simulink model "untitled1"  (R2019b)
settings: Solver=VariableStepAuto  StartTime=0.0  StopTime=10.0  RelTol=1e-3
libraries: neural x1015
(part 3 of 13)

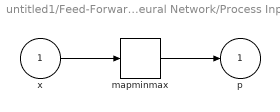
== system untitled1/Feed-Forward Neural Network/Process Input 1 ==
  x : Inport  PortDimensions=1001  SampleTime=0.1
      mask Display: e = 0.06;c1 = [120 230 180]/255;c2 = ([120 230 180]+0)/(256+128);c3 = ([120 230 180]+128)/(256+128);patch([0 1 1 0],[0 0 1 1],c1);patch([0 1 1 1-e 1-e 0+e],[0 0 1 1-e 0+e 0+e],c2);patch([0 0 1 1-e 0+e 0+e],[0 1 1 1-e 1-e 0+e],c3);plot([0 1 1 0 0],[0 0 1 1 0]);
  mapminmax : neural/Processing Functions/mapminmax  xmin=[2.22144146907918305089424393373;1.69636663439423740484812697105;1.23297861292478039274556067539;0.862805238425770837373818267224;0.640905167232490913242770602665;0.542648239835758716687053038186;0.499989859687834325985278383087;0.471682738351806851717640256538;0.441708721028247375262054674749;0.405589469414133874103356447449;0.363572961406947281481905065448;0.317837403618206004729529468023;0.271183905029315552859259241814;0.226267212986469901103703250556;0.185127098379413213002919746941;0.148992907869379576091262151749;0.118323297349533160249812624443;0.0929893241091522548824599425643;0.0724978614565823520354825859613;0.0561849446326162585418906303403;0.0433514048772383059349166956054;0.0333425112197407585989950007388;0.0255856435758149286519014253827;0.0196012832066613795767295869155;0.0149992993770703200717697711752;0.0114684591125998602834101802728;0.00876380997939582920275292110546;0.00669436749232934277115125709656;0.00511219525396657860361049330322;0.00390322240953329445758979154846;0.00297976937771365826129743581419;0.00227459017607360269169758382191;0.00173618904965629618046552007371;0.00132517309896925967321879014094;0.00101142975011124817627528038599;0.000771952018802877018566199751604;0.000589167891403684948307961644076;0.000449659595600714512460271965466;0.000343183150747135637392837281823;0.000261918520089536089635873228332;0.000199896507703293060693311433695;0.000152560939211198685070206004788;0.000116434295959401751447727380029;8.88624117084245315843077372975e-05;6.78195654303697574669801406699e-05;5.17596973061010750616697806414e-05;3.95028409195940653948764254011e-05;3.01484402164502406074302748307e-05;2.30091888936184349716967956212e-05;1.75605345651528290610698251895e-05;1.34021393389347518392386640618e-05;1.02284660433953875123894161625e-05;7.80632942694423752631651541867e-06;5.9577631396334876411405301333e-06;4.54694379857023389923100994969e-06;3.47021142741961576577854574344e-06;2.64845307330462529339589090871e-06;2.02128999980813789499856612808e-06;1.54264136030170991810883587142e-06;1.17733841377799769068357611801e-06;8.98540499805068613696913508437e-07;6.85762920246960633640428018493e-07;5.23371827044055577308708827877e-07;3.9943552062621165311482175457e-07;3.04847772073068712779070300531e-07;2.32658736929191716214830533589e-07;1.77564321489930699896303382956e-07;1.35516460234206524037474730915e-07;1.03425681560179677740212941285e-07;7.89341131179579374986825159727e-08;6.02422344982842236144380361137e-08;4.59766598110878228538888387155e-08;3.50892231862316141930009086216e-08;2.67799708225181090575254074827e-08;2.0438379242318883615440184274e-08;1.55984985123953711610413698811e-08;1.19047181170172037897621032361e-08;9.0856386374699334819759601674e-09;6.93412742240972023202099400077e-09;5.2921010176065205859308312672e-09;4.03891265656681822194088457654e-09;3.08248400609058246880866567259e-09;2.3525400965325377189293189564e-09;1.79545076429360288856288371172e-09;1.37028168710744951633642114633e-09;1.04579411955851293914931205499e-09;7.98146387741805226849521612081e-10;6.09142281703215494910457932155e-10;4.64895201804772115872786873727e-10;3.54806910828426062606473878575e-10;2.7078694900619653199012210042e-10;2.06663881817707040490304914005e-10;1.5772490134844833813048885824e-10;1.20375410324372701148682728947e-10;9.18697586638477560524196988315e-11;7.01145276943687131296985201443e-11;5.35108784964484267598601460541e-11;4.0839452243183072207030181867e-11;3.11689880456043393416875475612e-11;2.3787263156418867797298358586e-11;1.8154355532134926793189292714e-11;1.38559063951890901106595552137e-11;1.05745197122625699786323009374e-11;8.0702301306923715283465484549e-12;6.15957576748324364861555936397e-12;4.7009491616160335177358366425e-12;3.58762153705167870373903735483e-12;2.73867434463637770962224419494e-12;2.08923323030717043186819033893e-12;1.59465347728954653536516307967e-12;1.21726610580501247047877341321e-12;9.29865741569101279429360046436e-13;7.08734878795353993279140064677e-13 ...(+11488 chars)]  xmax=[2.82842712474619029094924371748;2.95205368510105126134135389293;2.97464691748655729597317076696;2.92820644854107703380918792391;2.8737880020283808057968144567;2.85480368143412155390592488402;2.88215601840531387978217026102;2.95559747403335348892028378032;3.07419534208398426144981385733;3.23783782353882498838970604993;3.4470168100608389316619195597;3.70249011389856264031550381333;4.00508598408322757933319735457;4.35569888348638656339062436018;4.75544470821087550405081856297;5.20588941109927016981373526505;5.70925826584193352175589097897;6.26857175092982554787113258499;6.88770373693512372170744129107;7.57138789847429993784544421942;8.32520376586147214936772797955;9.15556547519334706919380550971;10.069725413104837485889220261;11.0757970137798142928886591108;12.1827967261539829024741266039;13.400703567334117494169731799;14.7405345018458433514751959592;16.2144343100948233882263593841;17.8357791942788317385293339612;19.6192939265534036508142889943;21.5811828137186338949504715856;23.7392751336040177534414397087;26.1131860090993903611433779588;28.7244939481479555354326294037;31.5969365109892770249189197784;34.7566257844074684157931187656;38.2322855578563078893239435274;42.0555123163771753524997620843;46.2610623964519547257623344194;50.8871678982608415253707789816;55.9758842153384605921928596217;61.5734723339726954804973502178;67.7308193732964411992725217715;74.5039011862797337926167529076;81.9542912252368296321947127581;90.1497202967140651708177756518;99.1646922936791668234945973381;109.081161502091632087285688613;119.98927763887429875921952771;131.988205394159166417011874728;145.187025928063263791045756079;159.705728517338116034807171673;175.676301366809241244482109323;193.243931502040453551671816967;212.568324651315606388379819691;233.825157115852050537796458229;257.207672827055887410097057;282.928440109517168821184895933;311.221284120312361665128264576;342.343412532243291934719309211;376.577753785403388064878527075;414.235529163902526761376066133;455.659082080266443881555460393;501.224990288276217142993118614;551.347489317092936289554927498;606.482238248795283652725629508;667.130462073670400968694593757;733.843508281034473839099518955;807.22785910913614770834101364;887.950645020048568767379038036;976.745709522052607098885346204;1074.42028047425742443010676652;1181.86230852168296223680954427;1300.0485393738508719252422452;1430.05339331123582269356120378;1573.05873264235924580134451389;1730.36460590659521585621405393;1903.40106649725476017920300364;2093.74117314698014524765312672;2303.11529046167834167135879397;2533.42681950784617583849467337;2786.76950145863065699813887477;3065.44645160449363174848258495;3371.99109676494299492333084345;3709.19020644143711251672357321;4080.10922708558064186945557594;4488.12014979413834225852042437;4936.93216477355235838331282139;5430.62538125090759422164410353;5973.68791937599871744168922305;6571.05671131359849823638796806;7228.1623824449579842621460557;7950.97862068945414648624137044;8746.07648275839892448857426643;9620.68413103423881693743169308;10582.752544137661971035413444;11641.0277985514276224421337247;12805.1305784065698389895260334;14085.6436362472268228884786367;15494.2079998719491413794457912;17043.628799859143327921628952;18747.9916798450576607137918472;20622.7908478295648819766938686;22685.0699326125213701743632555;24953.5769258737745985854417086;27448.9346184611531498376280069;30193.8280803072702838107943535;33213.2108883379987673833966255;36534.5319771717986441217362881;40187.9851748889777809381484985;44206.7836923778741038404405117;48627.4620616156607866287231445;53490.208267777226865291595459;58839.2290945549466414377093315;64723.152004010444215964525938;71195.4672044114849995821714401;78315.0139248526393203064799309;86146.515317337907617911696434;94761.1668490716983797028660774;104237.283533978872583247721195;114661.011887376764207147061825;126127.113076114444993436336517;138739.824383725877851247787476;152613.80682209847145713865757;167875.187504308327334001660347 ...(+25362 chars)]  ymin=-1  ymax=1
      settings: SourceProductName=Deep Learning Toolbox
  p : Outport  PortDimensions=1001  SampleTime=0.1
      mask Display: e = 0.06;c1 = [120 230 180]/255;c2 = ([120 230 180]+0)/(256+128);c3 = ([120 230 180]+128)/(256+128);patch([0 1 1 0],[0 0 1 1],c1);patch([0 1 1 1-e 1-e 0+e],[0 0 1 1-e 0+e 0+e],c2);patch([0 0 1 1-e 0+e 0+e],[0 1 1 1-e 1-e 0+e],c3);plot([0 1 1 0 0],[0 0 1 1 0]);
  wires:
  x/1 -> mapminmax/1
  mapminmax/1 -> p/1
